simulink model "ANDGate"  (R2015a)
settings: Solver=ode45  StartTime=0.0  StopTime=0.01  RelTol=1e-3
libraries: powerlib x9
settings Model: Creator=asus  LastModifiedBy=asus

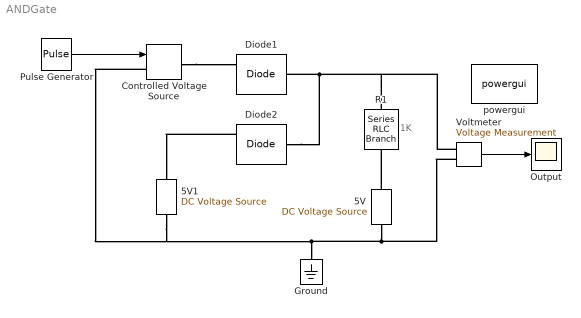
== system ANDGate ==
  note: 1K
  " 5V" : powerlib/Electrical Sources/DC Voltage Source  Amplitude=5  Measurements=Voltage
  " 5V1" : powerlib/Electrical Sources/DC Voltage Source  Amplitude=5  Measurements=Voltage
  Controlled Voltage Source : powerlib/Electrical Sources/Controlled Voltage Source  Initialize=off  Source_Type=AC  Amplitude=0  Phase=0  Frequency=0  Measurements=Voltage
  Diode1 : powerlib/Power Electronics/Diode  Ron=0.001  Lon=0  Vf=0.8  IC=0  UseSnubber=off  Rs=0  Cs=0  Measurements=on
  Diode2 : powerlib/Power Electronics/Diode  Ron=0.001  Lon=0  Vf=0.8  IC=0  UseSnubber=off  Rs=0  Cs=0  Measurements=on
  Ground : powerlib/Elements/Ground  LConnTagsString=a
  Output : Scope
      settings: YMin=0  YMax=6
  Pulse Generator : DiscretePulseGenerator  PulseType=Time based  Amplitude=4  Period=1e-3  PulseWidth=50
  R1 : powerlib/Elements/Series RLC Branch  LConnTagsString=__new0  RConnTagsString=__new0  BranchType=R  Resistance=1000  Inductance=1e-3  SetiL0=off  InitialCurrent=0  Capacitance=1e-6  Setx0=off  InitialVoltage=0  Measurements=None
  Voltmeter : powerlib/Measurements/Voltage Measurement  PhasorSimulation=off  OutputType=Complex  PSBequivalent=0
  powergui : powerlib/powergui  Priority=1  SimulationMode=Discrete  SolverType=Tustin/Backward Euler (TBE)  SampleTime=10e-6  frequency=60  SPID=off  DisableSnubberDevices=off  DisableRonSwitches=off  DisableVfSwitches=off  SwTol=0  DisplayEquations=off  Interpol=off  methode=off  Ts=100  FunctionMessages=off  echomessages=off  HookPort=off  EnableUseOfTLC=off  x0status=blocks  frequencyindice=0  Pbase=100e6  ErrMax=1e-4  Iterations=50  UnitsV=kV  UnitsW=MW  buscounter=0  RestoreLinks=warning  ResistiveCurrentMeasurement=off  Frange=[0:2:500]  Ylog=off  Xlog=on  ShowGrid=off  save=off  variable=ZData  structure=0  ZoomFFT=off  StartTime=0.0  cycles=1  DisplayStyle=1  fundamental=60  FreqAxis=off  MaxFrequency=1000  frequencyindicesteady=1  RmsSteady=1  display=off
  wires:
  Pulse Generator/1 -> Controlled Voltage Source/1
  Voltmeter/1 -> Output/1
  connections:
  Voltmeter/LConn2 -- " 5V"/LConn1 -- " 5V1"/LConn1 -- Controlled Voltage Source/LConn1 -- Ground/LConn1
  " 5V"/RConn1 -- R1/RConn1
  Diode2/LConn1 -- R1/LConn1 -- Voltmeter/LConn1 -- Diode1/LConn1
  Controlled Voltage Source/RConn1 -- Diode1/RConn1
  Diode2/RConn1 -- " 5V1"/RConn1
